simulink model "Simscape_Benchmark_Model"  (R2020b)
settings: Solver=ode45  StartTime=0.0  StopTime=10.0  RelTol=1e-8  AbsTol=1e-9
undefined symbols (not defined in the file): Bus, FSM, ISOL, Model, PMA, RWIsol, RWS, SA, SADM, slosh, X, Y, Z
libraries: sm_lib x159, nesl_utility x85, simulink x4
(part 6 of 6)

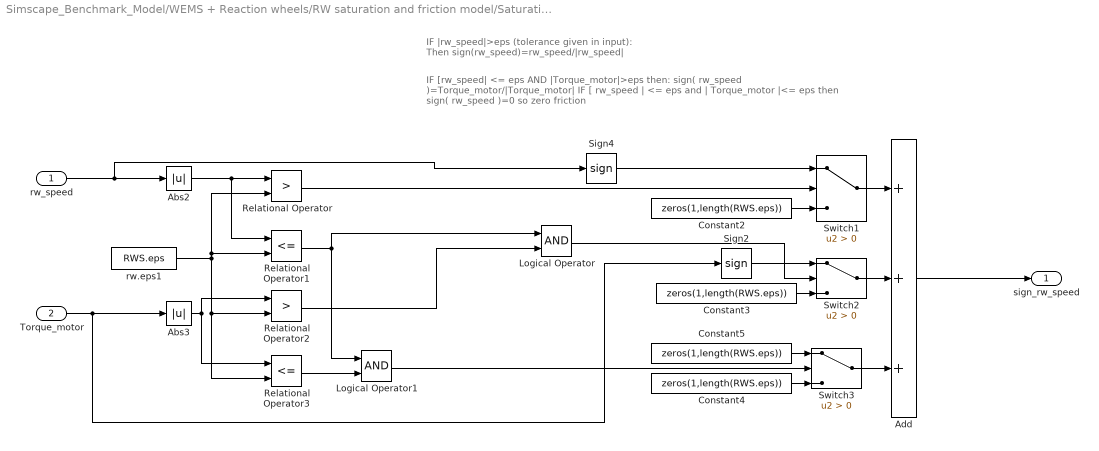
== system Simscape_Benchmark_Model/WEMS + Reaction wheels/RW saturation and friction model/Saturations + friction model + friction spikes/RW friction model/Friction model (torque)1/Computation of the sign of rw_speed ==
  note: IF [rw_speed| <= eps AND |Torque_motor|>eps then:
      | sign( rw_speed )=Torque_motor/|Torque_motor|
      |
      | IF [ rw_speed | <= eps and | Torque_motor |<= eps then sign( rw_speed )=0 so zero friction
  note: IF |rw_speed|>eps (tolerance given in input):
      | Then sign(rw_speed)=rw_speed/|rw_speed|
  rw_speed : Inport
  Torque_motor : Inport  Port=2
  Abs2 : Abs  SaturateOnIntegerOverflow=on
  Abs3 : Abs  SaturateOnIntegerOverflow=on
  Add : Sum  Inputs=+++
  Constant{2..5} (4 alike) : Constant  Value=zeros(1,length(RWS.eps))
  Logical Operator : Logic  AllPortsSameDT=off  OutDataTypeStr=boolean
  Logical Operator1 : Logic  AllPortsSameDT=off  OutDataTypeStr=boolean
  Relational Operator : RelationalOperator  Operator=>  OutDataTypeStr=boolean  ZeroCross=off  RndMeth=Nearest
  Relational Operator1 : RelationalOperator  Operator=<=  OutDataTypeStr=boolean  RndMeth=Nearest
  Relational Operator2 : RelationalOperator  Operator=>  OutDataTypeStr=boolean  ZeroCross=off  RndMeth=Nearest
  Relational Operator3 : RelationalOperator  Operator=<=  OutDataTypeStr=boolean  ZeroCross=off  RndMeth=Nearest
  Sign2 : Signum  ZeroCross=off
  Sign4 : Signum
  Switch1 : Switch  Criteria=u2 > Threshold  ZeroCross=off
  Switch2 : Switch  Criteria=u2 > Threshold  ZeroCross=off
  Switch3 : Switch  Criteria=u2 > Threshold  ZeroCross=off
  rw.eps1 : Constant  Value=RWS.eps
  sign_rw_speed : Outport  VectorParamsAs1DForOutWhenUnconnected=off
  wires:
  Logical Operator1/1 -> Switch3/2
  Logical Operator/1 -> Switch2/2
  Relational Operator3/1 -> Logical Operator1/2
  Relational Operator2/1 -> Logical Operator/2
  Abs3/1 -> Relational Operator3/1, Relational Operator2/1
  Relational Operator1/1 -> Logical Operator1/1, Logical Operator/1
  rw.eps1/1 -> Relational Operator/2, Relational Operator1/2, Relational Operator3/2, Relational Operator2/2
  Abs2/1 -> Relational Operator1/1, Relational Operator/1
  rw_speed/1 -> Sign4/1, Abs2/1
  Switch2/1 -> Add/2
  Constant5/1 -> Switch3/1
  Constant3/1 -> Switch2/3
  Sign4/1 -> Switch1/1
  Relational Operator/1 -> Switch1/2
  Switch1/1 -> Add/1
  Constant4/1 -> Switch3/3
  Constant2/1 -> Switch1/3
  Switch3/1 -> Add/3
  Sign2/1 -> Switch2/1
  Add/1 -> sign_rw_speed/1
  Torque_motor/1 -> Sign2/1, Abs3/1

== system Simscape_Benchmark_Model/WEMS + Reaction wheels/RW saturation and friction model/Saturations + friction model + friction spikes/RW friction model/Friction model (torque)1/Friction torque calculation ==
  note: IF |rw_speed|<=RWS.w_threshold then:
      |
      | Torque_stiction=-k_stiction*sign(rw_speed)
      |
      | otherwise Torque_stiction=0
  note: IF |rw_speed|>RWS.w_threshold then:
      |
      | Torque_Coulomb=-k_Coulomb*sign(rw_speed)
      |
      | otherwise Torque_Coulomb=0
  note: Torque_viscous=-k_viscous* rw_speed
  rw_speed : Inport
  sign_rw_speed : Inport  Port=2
  Abs : Abs  SaturateOnIntegerOverflow=on
  Gain : Gain  Gain=-1  SaturateOnIntegerOverflow=on  OutDataTypeStr=Inherit: Same as input  ParamDataTypeStr=Inherit: Same as input
  Gain1 : Gain  Gain=-1  SaturateOnIntegerOverflow=on  OutDataTypeStr=Inherit: Same as input  ParamDataTypeStr=Inherit: Same as input
  Gain2 : Gain  Gain=-1  SaturateOnIntegerOverflow=on  OutDataTypeStr=Inherit: Same as input  ParamDataTypeStr=Inherit: Same as input
  Switch : Switch  Threshold=RWS.w_threshold  ZeroCross=off  SaturateOnIntegerOverflow=on
  Switch2 : Switch  Threshold=RWS.w_threshold  ZeroCross=off  SaturateOnIntegerOverflow=on
  Torque_Coulomb=0 : Constant  Value=0
  Torque_stiction=0 : Constant  Value=0
  k_Coulomb : Gain  Gain=RWS.k_coulomb  SaturateOnIntegerOverflow=on  OutDataTypeStr=Inherit: Same as input  ParamDataTypeStr=Inherit: Same as input
  k_stiction : Gain  Gain=RWS.k_stiction  SaturateOnIntegerOverflow=on  OutDataTypeStr=Inherit: Same as input  ParamDataTypeStr=Inherit: Same as input
  k_viscous : Gain  Gain=RWS.k_viscous  SaturateOnIntegerOverflow=on  OutDataTypeStr=Inherit: Same as input  ParamDataTypeStr=Inherit: Same as input
  Torque_Coulomb : Outport  VectorParamsAs1DForOutWhenUnconnected=off
  Torque_stiction : Outport  Port=2  VectorParamsAs1DForOutWhenUnconnected=off
  Torque_viscous : Outport  Port=3  VectorParamsAs1DForOutWhenUnconnected=off
  wires:
  k_viscous/1 -> Torque_viscous/1
  Gain2/1 -> k_viscous/1
  Torque_stiction=0/1 -> Switch2/1
  k_stiction/1 -> Switch2/3
  Torque_Coulomb=0/1 -> Switch/3
  k_Coulomb/1 -> Switch/1
  Gain1/1 -> k_stiction/1
  Gain/1 -> k_Coulomb/1
  rw_speed/1 -> Gain2/1, Abs/1
  Abs/1 -> Switch2/2, Switch/2
  sign_rw_speed/1 -> Gain1/1, Gain/1
  Switch/1 -> Torque_Coulomb/1
  Switch2/1 -> Torque_stiction/1

== matlab function Simscape_Benchmark_Model/WEMS + Reaction wheels/RW saturation and friction model/Saturations + friction model + friction spikes/Spike generation RW2/Set_spike_duration ==
  data: uk input; uk_1 input; y output; counter input
function y = fcn(uk,uk_1,counter)

if uk==uk_1
y = counter+1;
else 
  y=0;
end

== matlab function Simscape_Benchmark_Model/WEMS + Reaction wheels/RW saturation and friction model/Saturations + friction model + friction spikes/Spike generation RW3/Set_spike_duration ==
  data: uk input; uk_1 input; y output; counter input
function y = fcn(uk,uk_1,counter)

if uk==uk_1
y = counter+1;
else 
  y=0;
end

== matlab function Simscape_Benchmark_Model/WEMS + Reaction wheels/RW saturation and friction model/Saturations + friction model + friction spikes/Spike generation RW4/Set_spike_duration ==
  data: uk input; uk_1 input; y output; counter input
function y = fcn(uk,uk_1,counter)

if uk==uk_1
y = counter+1;
else 
  y=0;
end

== matlab function Simscape_Benchmark_Model/WEMS + Reaction wheels/RW saturation and friction model/Saturations + friction model + friction spikes/Spike generation RW1/Set_spike_duration ==
  data: uk input; uk_1 input; y output; counter input
function y = fcn(uk,uk_1,counter)

if uk==uk_1
y = counter+1;
else 
  y=0;
end
